simulink model "variant_3_MRC_SimulationModel"  (R2015b)
settings: Solver=ode3  SolverMode=SingleTasking  StartTime=0.0  StopTime=inf  RelTol=1e-3
PreLoadFcn:
  | addLibrariesInPath('sim')
PostLoadFcn:
  | loadRobotParameters
StartFcn:
  | simApp = SimDisplay.getInstance;
  | simApp.reset;
  | simApp.TrackView.setup(double(SitesPositions), ObstaclesPositions,ObstaclesVertices,ObstaclesEdges);
undefined symbols (not defined in the file): AngularSpeed, AxleLength, do_one_run, EncL_init, EncR_init, EncRes, lcam, motorL, motorR, motorX, ObstaclesEdges, ObstaclesVertices, pcam, SitesPositions, startPos, TauMotor, theta0, Ts, WheelRadius
libraries: simulink x2, realtime_pacer_lib x1, cstblocks x1, simulink_extras x1
(part 2 of 3)

== stateflow chart variant_3_MRC_SimulationModel/InputProcessing/Brain ==
  state Mapping [parallel]
    settings: executionOrder=2
    state Gestion_Rien
      %Entrée dans cet état si la camera ni détecte ni cible ni obstacle
      %Entrée dans un des blocs suivant l'orientation du robot : Nord, Nord-Est,...
      %Les blocs devant le robot (dans le champ de vision de la caméra) sont mis à jour à rien
      entry:
      ajout_cible_nv=false;
      ajout_cible_v=false;
      fin=false;
      Coef_bord_x=0;
      Coef_bord_y=0;
      bord = false;
      state Nord_Est
        entry: %-22.5
        % 0.7 pour sin(45°)
        state Obstacle
          entry:
          Carte(Distance_max_x-1, Distance_max_y+1)=3;
        state Bord_gauche
          entry:
          Coef_bord_y=-2;
          %Coef_bord_x=0;
        state Bord_droit
          entry:
          Coef_bord_x=+2;
        state Distance
          entry:
          Distance_max_x=xy_carte(1)-round(distObsM/10)-1;
          Distance_max_y=xy_carte(2)+round(distObsM/10)+1;
        state x_max
          entry:
          Distance_max_x = 2;
        state y_max
          entry:
          Distance_max_y = 29;
        state Mise_a_jour_carte
          entry:
          Carte(xy_carte(1)-1, xy_carte(2)+1)=4;
          Carte(xy_carte(1)-2, xy_carte(2)+2)=4;
          Carte(Distance_max_x+1+Coef_bord_x:xy_carte(1)-3+Coef_bord_x, xy_carte(2)+3+Coef_bord_y:Distance_max_y-1+Coef_bord_y)=4;
        state Fin
          entry:
          fin=true;
        state Bord2
          entry:
          Carte(Distance_max_x:xy_carte(1)-3, Distance_max_y-3:Distance_max_y-2)=4;
          Carte(Distance_max_x+2:Distance_max_x+3, xy_carte(2)+3:Distance_max_y)=4;
        (default) -> Bord_gauche [order 2] : [orientation > -28]
        (default) -> Bord_droit [order 1] : [orientation < -62 ]
        (default) -> Distance [order 3] : [orientation <= -28 && orientation >= -62]
        Mise_a_jour_carte -> Obstacle [order 1] : [distObsM < 60 && bord]
        Obstacle -> Fin : [1]
        Bord_droit -> Distance
        Bord_gauche -> Distance
        Distance -> x_max [order 1] : [Distance_max_x < 2]
        Distance -> y_max [order 2] : [Distance_max_y > 29]
        Distance -> Mise_a_jour_carte [order 3] : [Distance_max_x > 1 && Distance_max_y < 30]
        y_max -> x_max [order 2] : [Distance_max_x < 2]
        x_max -> y_max [order 1] : [Distance_max_y > 29]
        y_max -> Mise_a_jour_carte [order 1] : [1]
        x_max -> Mise_a_jour_carte [order 2] : [1]
        Mise_a_jour_carte -> Bord2 [order 3] : [bord==false]
        Mise_a_jour_carte -> Fin [order 2] : [distObsM == 60 && bord]
        Bord2 -> Fin : [1]
      state Nord_Ouest
        state Bord_gauche1
          entry:
          Coef_bord_x=+2;
          bord = true;
        state Bord_droit1
          entry:
          Coef_bord_y=+2;
          bord=true;
        state Obstacle1
          entry:
          Carte(Distance_max_x-1, Distance_max_y-1)=3;
        state Distance1
          entry:
          Distance_max_x=xy_carte(1)-round(distObsM/10)-1;
          Distance_max_y=xy_carte(2)-round(distObsM/10)-1;
        state y_max1
          entry:
          Distance_max_y = 2;
        state x_max1
          entry:
          Distance_max_x = 2;
        state Mise_a_jour_carte1
          entry:
          Carte(xy_carte(1)-1, xy_carte(2)-1)=4;
          Carte(xy_carte(1)-2, xy_carte(2)-2)=4;
          Carte(Distance_max_x+1+Coef_bord_x:xy_carte(1)-3+Coef_bord_x, Distance_max_y+1+Coef_bord_y:xy_carte(2)-3+Coef_bord_y)=4;
        state Fin1
          entry:
          fin=true;
        state Bord1
          entry:
          Carte(Distance_max_x:xy_carte(1)+3, Distance_max_y+2:Distance_max_y+3)=4;
          Carte(Distance_max_x+2:Distance_max_x+3, Distance_max_y:xy_carte(2)+3)=4;
        (default) -> Mapping.Gestion_Rien.Nord_Ouest.Bord_gauche1 [order 1] : [orientation > -28]
        (default) -> Mapping.Gestion_Rien.Nord_Ouest.Bord_droit1 [order 2] : [orientation < -53 ]
        (default) -> Mapping.Gestion_Rien.Nord_Ouest.Distance1 [order 3] : [orientation <= -28 && orientation >= -53]
        Mapping.Gestion_Rien.Nord_Ouest.Bord_droit1 -> Mapping.Gestion_Rien.Nord_Ouest.Distance1
        Mapping.Gestion_Rien.Nord_Ouest.Bord_gauche1 -> Mapping.Gestion_Rien.Nord_Ouest.Distance1
        Mapping.Gestion_Rien.Nord_Ouest.Distance1 -> Mapping.Gestion_Rien.Nord_Ouest.x_max1 [order 1] : [Distance_max_x < 2]
        Mapping.Gestion_Rien.Nord_Ouest.Mise_a_jour_carte1 -> Mapping.Gestion_Rien.Nord_Ouest.Obstacle1 [order 1] : [distObsM < 60 && bord]
        Mapping.Gestion_Rien.Nord_Ouest.Obstacle1 -> Mapping.Gestion_Rien.Nord_Ouest.Fin1 : [1]
        Mapping.Gestion_Rien.Nord_Ouest.Distance1 -> Mapping.Gestion_Rien.Nord_Ouest.y_max1 [order 2] : [Distance_max_y < 2]
        Mapping.Gestion_Rien.Nord_Ouest.Distance1 -> Mapping.Gestion_Rien.Nord_Ouest.Mise_a_jour_carte1 [order 3] : [Distance_max_x > 1 && Distance_max_y > 1]
        Mapping.Gestion_Rien.Nord_Ouest.y_max1 -> Mapping.Gestion_Rien.Nord_Ouest.x_max1 [order 2] : [Distance_max_x < 2]
        Mapping.Gestion_Rien.Nord_Ouest.x_max1 -> Mapping.Gestion_Rien.Nord_Ouest.y_max1 [order 1] : [Distance_max_y < 2]
        Mapping.Gestion_Rien.Nord_Ouest.y_max1 -> Mapping.Gestion_Rien.Nord_Ouest.Mise_a_jour_carte1 [order 1] : [1]
        Mapping.Gestion_Rien.Nord_Ouest.x_max1 -> Mapping.Gestion_Rien.Nord_Ouest.Mise_a_jour_carte1 [order 2] : [1]
        Mapping.Gestion_Rien.Nord_Ouest.Mise_a_jour_carte1 -> Mapping.Gestion_Rien.Nord_Ouest.Bord1 [order 3] : [bord==false]
        Mapping.Gestion_Rien.Nord_Ouest.Mise_a_jour_carte1 -> Mapping.Gestion_Rien.Nord_Ouest.Fin1 [order 2] : [distObsM == 60 && bord]
        Mapping.Gestion_Rien.Nord_Ouest.Bord1 -> Mapping.Gestion_Rien.Nord_Ouest.Fin1 : [1]
      state Nord
        entry:
        state Distance2
          entry:
          Distance_max=xy_carte(1)-round(distObsM/10);
        state y_max2
          entry:
          Distance_max = 1;
        state Mise_a_jour_carte2
          entry:
          Carte(Distance_max:xy_carte(1), xy_carte(2))=4;
          Carte(Distance_max:xy_carte(1)-1, xy_carte(2)-1:xy_carte(2)+1)=4;
          Carte(Distance_max:xy_carte(1)-2, xy_carte(2)-2:xy_carte(2)+2)=4;
        state Obstacle2
          entry:
          Carte(Distance_max, xy_carte(2)-1:xy_carte(2)+1)=3;
        state Fin2
          entry:
          fin=true;
        (default) -> Mapping.Gestion_Rien.Nord.Distance2
        Mapping.Gestion_Rien.Nord.Distance2 -> Mapping.Gestion_Rien.Nord.y_max2 [order 1] : [Distance_max < 1]
        Mapping.Gestion_Rien.Nord.y_max2 -> Mapping.Gestion_Rien.Nord.Mise_a_jour_carte2 : [1]
        Mapping.Gestion_Rien.Nord.Distance2 -> Mapping.Gestion_Rien.Nord.Mise_a_jour_carte2 [order 2] : [Distance_max > 0]
        Mapping.Gestion_Rien.Nord.Mise_a_jour_carte2 -> Mapping.Gestion_Rien.Nord.Obstacle2 [order 1] : [distObsM < 60]
        Mapping.Gestion_Rien.Nord.Obstacle2 -> Mapping.Gestion_Rien.Nord.Fin2 : [1]
        Mapping.Gestion_Rien.Nord.Mise_a_jour_carte2 -> Mapping.Gestion_Rien.Nord.Fin2 [order 2] : [distObsM == 60]
      state Ouest
        state Distance2
          entry:
          Distance_max=xy_carte(2)-round(distObsM/10);
        state y_max2
          entry:
          Distance_max = 1;
        state Obstacle2
          entry:
          Carte(xy_carte(1)-1:xy_carte(1)+1, Distance_max)=3;
        state Mise_a_jour_carte2
          entry:
          Carte(xy_carte(1), Distance_max:xy_carte(2))=4;
          Carte(xy_carte(1)-1:xy_carte(1)+1, Distance_max:xy_carte(2)-1)=4;
          Carte(xy_carte(1)-2:xy_carte(1)+2, Distance_max:xy_carte(2)-3)=4;
        state Fin2
          entry:
          fin=true;
        (default) -> Mapping.Gestion_Rien.Ouest.Distance2
        Mapping.Gestion_Rien.Ouest.Distance2 -> Mapping.Gestion_Rien.Ouest.y_max2 [order 1] : [Distance_max < 1]
        Mapping.Gestion_Rien.Ouest.y_max2 -> Mapping.Gestion_Rien.Ouest.Mise_a_jour_carte2 : [1]
        Mapping.Gestion_Rien.Ouest.Distance2 -> Mapping.Gestion_Rien.Ouest.Mise_a_jour_carte2 [order 2] : [Distance_max > 0]
        Mapping.Gestion_Rien.Ouest.Mise_a_jour_carte2 -> Mapping.Gestion_Rien.Ouest.Obstacle2 [order 1] : [distObsM < 60]
        Mapping.Gestion_Rien.Ouest.Obstacle2 -> Mapping.Gestion_Rien.Ouest.Fin2 : [1]
        Mapping.Gestion_Rien.Ouest.Mise_a_jour_carte2 -> Mapping.Gestion_Rien.Ouest.Fin2 [order 2] : [distObsM == 60]
      state Est
        entry:
        state Distance1
          entry:
          Distance_max=xy_carte(2)+round(distObsM/10);
        state y_max1
          entry:
          Distance_max = 30;
        state Obstacle1
          entry:
          Carte(xy_carte(1)-1:xy_carte(1)+1, Distance_max)=3;
        state Mise_a_jour_carte1
          entry:
          Carte(xy_carte(1), xy_carte(2):Distance_max)=4;
          Carte(xy_carte(1)-1:xy_carte(1)+1, xy_carte(2)+1:Distance_max)=4;
          Carte(xy_carte(1)-2:xy_carte(1)+2, xy_carte(2)+3:Distance_max)=4;
        state Fin1
          entry:
          fin=true;
        (default) -> Mapping.Gestion_Rien.Est.Distance1
        Mapping.Gestion_Rien.Est.Distance1 -> Mapping.Gestion_Rien.Est.y_max1 [order 1] : [Distance_max > 30]
        Mapping.Gestion_Rien.Est.y_max1 -> Mapping.Gestion_Rien.Est.Mise_a_jour_carte1 : [1]
        Mapping.Gestion_Rien.Est.Distance1 -> Mapping.Gestion_Rien.Est.Mise_a_jour_carte1 [order 2] : [Distance_max < 31]
        Mapping.Gestion_Rien.Est.Mise_a_jour_carte1 -> Mapping.Gestion_Rien.Est.Obstacle1 [order 1] : [distObsM < 60]
        Mapping.Gestion_Rien.Est.Obstacle1 -> Mapping.Gestion_Rien.Est.Fin1 : [1]
        Mapping.Gestion_Rien.Est.Mise_a_jour_carte1 -> Mapping.Gestion_Rien.Est.Fin1 [order 2] : [distObsM == 60]
      state Sud
        entry:
        state Distance2
          entry:
          Distance_max=xy_carte(1)+round(distObsM/10);
        state y_max2
          entry:
          Distance_max = 30;
        state Obstacle2
          entry:
          Carte(Distance_max, xy_carte(2)-1:xy_carte(2)+1)=3;
        state Mise_a_jour_carte2
          entry:
          Carte(xy_carte(1):Distance_max, xy_carte(2))=4;
          Carte(xy_carte(1)+1:Distance_max, xy_carte(2)-1:xy_carte(2)+1)=4;
          Carte(xy_carte(1)+2:Distance_max, xy_carte(2)-2:xy_carte(2)+2)=4;
        state Fin2
          entry:
          fin=true;
        (default) -> Mapping.Gestion_Rien.Sud.Distance2
        Mapping.Gestion_Rien.Sud.Distance2 -> Mapping.Gestion_Rien.Sud.y_max2 [order 1] : [Distance_max > 30]
        Mapping.Gestion_Rien.Sud.y_max2 -> Mapping.Gestion_Rien.Sud.Mise_a_jour_carte2 : [1]
        Mapping.Gestion_Rien.Sud.Distance2 -> Mapping.Gestion_Rien.Sud.Mise_a_jour_carte2 [order 2] : [Distance_max < 31]
        Mapping.Gestion_Rien.Sud.Mise_a_jour_carte2 -> Mapping.Gestion_Rien.Sud.Obstacle2 [order 1] : [distObsM < 60]
        Mapping.Gestion_Rien.Sud.Obstacle2 -> Mapping.Gestion_Rien.Sud.Fin2 : [1]
        Mapping.Gestion_Rien.Sud.Mise_a_jour_carte2 -> Mapping.Gestion_Rien.Sud.Fin2 [order 2] : [distObsM == 60]
      state Sud_Ouest
        entry:
        state Bord_gauche2
          entry:
          Coef_bord_y=+2;
          bord=true;
        state Bord_droit2
          entry:
          Coef_bord_x=-2;
          bord=true;
        state Obstacle2
          entry:
          Carte(Distance_max_x+1, Distance_max_y-1)=3;
        state Distance2
          entry:
          Distance_max_x=xy_carte(1)+round(distObsM/10)+1;
          Distance_max_y=xy_carte(2)-round(distObsM/10)-1;
        state x_max2
          entry:
          Distance_max_x = 29;
        state y_max2
          entry:
          Distance_max_y = 2;
        state Mise_a_jour_carte2
          entry:
          Carte(xy_carte(1)+1, xy_carte(2)-1)=4;
          Carte(xy_carte(1)+2, xy_carte(2)-2)=4;
          Carte(xy_carte(1)+3+Coef_bord_x:Distance_max_x-1+Coef_bord_x, Distance_max_y+1+Coef_bord_y:xy_carte(2)-3+Coef_bord_y)=4;
        state Fin2
          entry:
          fin=true;
        state Bord1
          entry:
          Carte(xy_carte(1)+3:Distance_max_x, Distance_max_y-3:Distance_max_y-2)=4;
          Carte(Distance_max_x+2:Distance_max_x+3, Distance_max_y:xy_carte(2)-3)=4;
        (default) -> Bord_gauche2 [order 1] : [orientation > 98]
        (default) -> Bord_droit2 [order 2] : [orientation < 152 ]
        (default) -> Mapping.Gestion_Rien.Sud_Ouest.Distance2 [order 3] : [orientation <= 98 && orientation >= 152]
        Bord_droit2 -> Mapping.Gestion_Rien.Sud_Ouest.Distance2
        Bord_gauche2 -> Mapping.Gestion_Rien.Sud_Ouest.Distance2
        Mapping.Gestion_Rien.Sud_Ouest.Mise_a_jour_carte2 -> Mapping.Gestion_Rien.Sud_Ouest.Obstacle2 [order 1] : [distObsM < 60]
        Mapping.Gestion_Rien.Sud_Ouest.Obstacle2 -> Mapping.Gestion_Rien.Sud_Ouest.Fin2 : [1]
        Mapping.Gestion_Rien.Sud_Ouest.Distance2 -> x_max2 [order 1] : [Distance_max_x > 29]
        Mapping.Gestion_Rien.Sud_Ouest.Distance2 -> Mapping.Gestion_Rien.Sud_Ouest.y_max2 [order 2] : [Distance_max_y < 2]
        Mapping.Gestion_Rien.Sud_Ouest.Distance2 -> Mapping.Gestion_Rien.Sud_Ouest.Mise_a_jour_carte2 [order 3] : [Distance_max_x < 30 && Distance_max_y > 1]
        Mapping.Gestion_Rien.Sud_Ouest.y_max2 -> x_max2 [order 2] : [Distance_max_x > 29]
        Mapping.Gestion_Rien.Sud_Ouest.y_max2 -> Mapping.Gestion_Rien.Sud_Ouest.Mise_a_jour_carte2 [order 1] : [1]
        x_max2 -> Mapping.Gestion_Rien.Sud_Ouest.y_max2 [order 1] : [Distance_max_y < 2]
        x_max2 -> Mapping.Gestion_Rien.Sud_Ouest.Mise_a_jour_carte2 [order 2] : [1]
        Mapping.Gestion_Rien.Sud_Ouest.Bord1 -> Mapping.Gestion_Rien.Sud_Ouest.Fin2 : [1]
        Mapping.Gestion_Rien.Sud_Ouest.Mise_a_jour_carte2 -> Mapping.Gestion_Rien.Sud_Ouest.Fin2 [order 2] : [distObsM == 60 && bord]
        Mapping.Gestion_Rien.Sud_Ouest.Mise_a_jour_carte2 -> Mapping.Gestion_Rien.Sud_Ouest.Bord1 [order 3] : [bord==false]
      state Sud_Est
        entry:
        state Bord_gauche1
          entry:
          Coef_bord_x=-2;
          bord=true;
        state Bord_droit1
          entry:
          Coef_bord_y=-2;
          bord=true;
        state Distance1
          entry:
          Distance_max_x=xy_carte(1)+round(distObsM/10)+1;
          Distance_max_y=xy_carte(2)+round(distObsM/10)+1;
        state x_max1
          entry:
          Distance_max_x = 29;
        state y_max1
          entry:
          Distance_max_y = 29;
        state Obstacle1
          entry:
          Carte(Distance_max_x+1, Distance_max_y+1)=3;
        state Mise_a_jour_carte1
          entry:
          Carte(xy_carte(1)+1, xy_carte(2)+1)=4;
          Carte(xy_carte(1)+2, xy_carte(2)+2)=4;
          Carte(xy_carte(1)+3+Coef_bord_x:Distance_max_x-1+Coef_bord_x, xy_carte(2)+3+Coef_bord_y:Distance_max_y-1+Coef_bord_y)=4;
        state Fin1
          entry:
          fin=true;
        state Bord
          entry:
          Carte(xy_carte(1)+3:Distance_max_x, Distance_max_y-3:Distance_max_y-2)=4;
          Carte(Distance_max_x-3:Distance_max_x-2, xy_carte(2)+3:Distance_max_y)=4;
        (default) -> Mapping.Gestion_Rien.Sud_Est.Bord_gauche1 [order 2] : [orientation > -98]
        (default) -> Mapping.Gestion_Rien.Sud_Est.Bord_droit1 [order 3] : [orientation < -152 ]
        (default) -> Mapping.Gestion_Rien.Sud_Est.Distance1 [order 1] : [orientation <= -98 && orientation >= -152]
        Mapping.Gestion_Rien.Sud_Est.Bord_droit1 -> Mapping.Gestion_Rien.Sud_Est.Distance1
        Mapping.Gestion_Rien.Sud_Est.Bord_gauche1 -> Mapping.Gestion_Rien.Sud_Est.Distance1
        Mapping.Gestion_Rien.Sud_Est.Distance1 -> Mapping.Gestion_Rien.Sud_Est.x_max1 [order 1] : [Distance_max_x > 29]
        Mapping.Gestion_Rien.Sud_Est.Distance1 -> Mapping.Gestion_Rien.Sud_Est.y_max1 [order 2] : [Distance_max_y > 29]
        Mapping.Gestion_Rien.Sud_Est.Distance1 -> Mapping.Gestion_Rien.Sud_Est.Mise_a_jour_carte1 [order 3] : [Distance_max_x < 30 && Distance_max_y < 30]
        Mapping.Gestion_Rien.Sud_Est.x_max1 -> Mapping.Gestion_Rien.Sud_Est.y_max1 [order 1] : [Distance_max_y > 29]
        Mapping.Gestion_Rien.Sud_Est.y_max1 -> Mapping.Gestion_Rien.Sud_Est.Mise_a_jour_carte1 [order 1] : [1]
        Mapping.Gestion_Rien.Sud_Est.y_max1 -> Mapping.Gestion_Rien.Sud_Est.x_max1 [order 2] : [Distance_max_x > 29]
        Mapping.Gestion_Rien.Sud_Est.Mise_a_jour_carte1 -> Mapping.Gestion_Rien.Sud_Est.Obstacle1 [order 1] : [distObsM < 60]
        Mapping.Gestion_Rien.Sud_Est.x_max1 -> Mapping.Gestion_Rien.Sud_Est.Mise_a_jour_carte1 [order 2] : [1]
        Mapping.Gestion_Rien.Sud_Est.Obstacle1 -> Mapping.Gestion_Rien.Sud_Est.Fin1 : [1]
        Mapping.Gestion_Rien.Sud_Est.Mise_a_jour_carte1 -> Bord [order 3] : [bord==false]
        Mapping.Gestion_Rien.Sud_Est.Mise_a_jour_carte1 -> Mapping.Gestion_Rien.Sud_Est.Fin1 [order 2] : [distObsM == 60 && bord]
        Bord -> Mapping.Gestion_Rien.Sud_Est.Fin1 : [1]
      (default) -> Nord [order 1] : [(orientation>-18) && (orientation < 18)]
      (default) -> Nord_Ouest [order 8] : [(orientation>=18) && (orientation <= 72)]
      (default) -> Nord_Est [order 2] : [(orientation >=-72) && (orientation <= -18)]
      (default) -> Est [order 3] : [(orientation>-108) && (orientation < -72)]
      (default) -> Ouest [order 4] : [(orientation>72) && (orientation < 108)]
      (default) -> Sud_Ouest [order 7] : [(orientation>=108) && (orientation <= 162)]
      (default) -> Sud [order 6] : [(orientation>162) || (orientation < -162)]
      (default) -> Sud_Est [order 5] : [(orientation >= -162) && (orientation <= -108)]
    state init
      entry:
      % Initialisation de la carte : dimension : 30*30
      Carte=zeros(30,30); % Init à Inconnu
      % Initialisations des bords de la carte à obstacle
      Carte(:,1)=zeros(30,1)+3;
      Carte(:,30)=zeros(30,1)+3;
      Carte(1,:)=zeros(30,1)+3;
      Carte(30,:)=zeros(30,1)+3;
      % Initialisation de la position de départ à rien
      Carte(25,5)=4
      % Code :
      % 0 : Inconnu
      % 1 : Cible non visitée
      % 2 : Cible visitée
      % 3 : Obstacle
      % 4 : Rien
    state X_moins
      entry:
      Carte(2:xy_carte(1), xy_carte(2))=4;
    state Y_moins
      entry:
      Carte(xy_carte(1), 2:xy_carte(2))=4;
    state X_plus
      entry:
      Carte(xy_carte(1):29, xy_carte(2))=4;
    state Y_plus
      entry:
      Carte(xy_carte(1), xy_carte(2):29)=4;
    state XY_moins
      entry:
      Carte(2:xy_carte(1), 2:xy_carte(2))=4;
    state XY_moins1
      entry:
      Carte(xy_carte(1):29, xy_carte(2):29)=4;
    state Ajout_cible_non_visitee
      entry:
      Carte(30-round(cible_en_vue(2)/10), round(cible_en_vue(1)/10)) = 1;
    state Ajout_cible_visitee
      entry:
      %Carte(30-round(cible(2,num_cible)/10), round(cible(1,num_cible)/10)) = 2;
      Carte(xy_carte(1),xy_carte(2))=2;
    (default) -> Mapping.init
    Mapping.init -> Gestion_Rien : [1]
    Gestion_Rien -> Gestion_Rien [order 5] : [~ajout_cible_nv && ~ajout_cible_v && fin && xy_carte(1) >= 4 && xy_carte(2) >= 4 ...
        | && xy_carte(1) <= 26 && xy_carte(2) <= 26]
    Gestion_Rien -> X_moins [order 9] : [xy_carte(1) < 4]
    XY_moins -> X_moins [order 3] : [xy_carte(2) >= 4]
    X_moins -> Gestion_Rien : [xy_carte(1) >= 4]
    Gestion_Rien -> Y_moins [order 7] : [xy_carte(2) < 4]
    XY_moins -> Y_moins [order 2] : [xy_carte(1) >= 4]
    Y_moins -> Gestion_Rien : [xy_carte(2) >= 4]
    Gestion_Rien -> X_plus [order 8] : [xy_carte(1) > 26]
    XY_moins1 -> X_plus [order 3] : [xy_carte(2) <= 26]
    X_plus -> Gestion_Rien : [xy_carte(1)<=26]
    Gestion_Rien -> Y_plus [order 6] : [xy_carte(2) > 26]
    XY_moins1 -> Y_plus [order 2] : [xy_carte(1) <= 26]
    Y_plus -> Gestion_Rien : [xy_carte(2) <= 26]
    Gestion_Rien -> XY_moins [order 4] : [xy_carte(2) < 4 && xy_carte(1) < 4]
    XY_moins -> Gestion_Rien [order 1] : [xy_carte(2) >= 4 && xy_carte(1) >= 4]
    Gestion_Rien -> XY_moins1 [order 3] : [xy_carte(2) >26 && xy_carte(1) > 26]
    XY_moins1 -> Gestion_Rien [order 1] : [xy_carte(2) <= 26 && xy_carte(1) <= 26]
    Gestion_Rien -> Ajout_cible_non_visitee [order 1] : [ajout_cible_nv]
    Ajout_cible_non_visitee -> Gestion_Rien : [1]
    Ajout_cible_visitee -> Gestion_Rien : [1]
    Gestion_Rien -> Ajout_cible_visitee [order 2] : [ajout_cible_v]
  state condToStop =StopToTurn(quadrantD,quadrantF,signeA) [function]
    (default) -> (junction 1363)
    (junction 1363) -> (junction 1359) [order 4]
    (junction 1363) -> (junction 1376) [order 1] : [quadrantD==4]
    (junction 1363) -> (junction 1390) [order 3] : [quadrantD==2]
    (junction 1363) -> (junction 1318) [order 2] : [quadrantD==1]
    (junction 1376) -> (junction 1326) [order 1] : [quadrantF==4]
    (junction 1318) -> (junction 1514) [order 1] : [quadrantF==3]
    (junction 1376) -> (junction 1130) [order 4]
    (junction 1318) -> (junction 1452) [order 4]
    (junction 1376) -> (junction 1151) [order 2] : [quadrantF==1]
    (junction 1318) -> (junction 1523) [order 2] : [quadrantF==4]
    (junction 1376) -> (junction 1411) [order 3] : [quadrantF==2]
    (junction 1318) -> (junction 1354) [order 3] : [quadrantF==1]
    (junction 1359) -> (junction 1459) [order 1] : [quadrantF==1]
    (junction 1359) -> (junction 1458) [order 4]
    (junction 1359) -> (junction 1517) [order 2] : [quadrantF==4]
    (junction 1390) -> (junction 1399) [order 1] : [quadrantF==4]
    (junction 1390) -> (junction 1421) [order 4]
    (junction 1359) -> (junction 1451) [order 3] : [quadrantF==3]
    (junction 1390) -> (junction 1340) [order 2] : [quadrantF==1]
    (junction 1390) -> (junction 1528) [order 3] : [quadrantF==2]
    (junction 1411) -> (junction 1188) [order 2]
    (junction 1354) -> (junction 1495) [order 2]
    (junction 1326) -> (junction 1520) [order 1] : [signeA==1]
    (junction 1514) -> (junction 1396) [order 1] : [signeA==1]
    (junction 1411) -> (junction 1350) [order 1] : [signeA==1]
    (junction 1354) -> (junction 1327) [order 1] : [signeA==1]
    (junction 1326) -> (junction 1454) [order 2]
    (junction 1514) -> (junction 1432) [order 2]
    (junction 1151) -> (junction 1478) : {condToStop=2;}
    (junction 1130) -> (junction 1337) : {condToStop=1;}
    (junction 1523) -> (junction 1362) : {condToStop=1;}
    (junction 1452) -> (junction 1409) : {condToStop=2;}
    (junction 1451) -> (junction 1191) [order 2]
    (junction 1459) -> (junction 1391) [order 1] : [signeA==1]
    (junction 1451) -> (junction 1494) [order 1] : [signeA==1]
    (junction 1459) -> (junction 1128) [order 2]
    (junction 1517) -> (junction 1392) : {condToStop=2;}
    (junction 1458) -> (junction 1336) : {condToStop=3;}
    (junction 1528) -> (junction 1335) [order 2]
    (junction 1399) -> (junction 1164) [order 1] : [signeA==1]
    (junction 1528) -> (junction 1502) [order 1] : [signeA==1]
    (junction 1399) -> (junction 1488) [order 2]
    (junction 1340) -> (junction 1445) : {condToStop=1;}
    (junction 1421) -> (junction 1308) : {condToStop=4;}
    (junction 1520) -> (junction 1472) : {condToStop=1;}
    (junction 1350) -> (junction 1170) : {condToStop=3;}
    (junction 1188) -> (junction 1329) : {condToStop=2;}
    (junction 1396) -> (junction 1526) : {condToStop=1;}
    (junction 1327) -> (junction 1169) : {condToStop=1;}
    (junction 1495) -> (junction 1507) : {condToStop=2;}
    (junction 1454) -> (junction 1131) : {condToStop=2;}
    (junction 1432) -> (junction 1119) : {condToStop=4;}
    (junction 1391) -> (junction 1497) : {condToStop=3;}
    (junction 1494) -> (junction 1374) : {condToStop=1;}
    (junction 1191) -> (junction 1174) : {condToStop=2;}
    (junction 1128) -> (junction 1491) : {condToStop=2;}
    (junction 1164) -> (junction 1140) : {condToStop=1;}
    (junction 1502) -> (junction 1165) : {condToStop=1;}
    (junction 1335) -> (junction 1156) : {condToStop=2;}
    (junction 1488) -> (junction 1435) : {condToStop=4;}
  state GoTo [parallel]
    settings: executionOrder=4
    state To
      entry:
      Cmd.Mode = EMode.SPEED;
      Cmd.Angle=single(0);
      Cmd.Position=single(0);
      if ((Target==3 || Target==4 || Target==5) && next)
      xyf=cible_en_vue
      else
      xyf=[(I_col*10);(300-I_row*10)]
      end
      %xyfp=xyf;
      xyi=[xy(1);xy(2)];
      distance=sqrt((xyf(2)-xy(2))^2+(xyf(1)-xy(1))^2);
      orientationI=orientation;
      angle=acosd(abs(xyf(2)-xy(2))/distance);
      v=0;
      (default) -> (junction 1146)
      (junction 1146) -> (junction 1189) [order 2]
      (junction 1189) -> (junction 1173) [order 1] : [xyf(1)>=xy(1)]
      (junction 1146) -> (junction 1313) [order 1] : [xyf(2)>=xy(2)]
      (junction 1189) -> (junction 1324) [order 2] : {anglef=180-angle;}%quadrant II
      (junction 1173) -> (junction 1510) : {anglef=-(180-angle);}%quadrant III
      (junction 1324) -> (junction 1510)
      (junction 1510) -> (junction 1518)
      (junction 1313) -> (junction 1135) [order 1] : [xyf(1)>xy(1)]
      (junction 1313) -> (junction 1430) [order 2] : {anglef=angle;}%quadrant I
      (junction 1135) -> (junction 1518) : {anglef=-angle;} %quadrant IV
      (junction 1518) -> (junction 1430)
      (junction 1430) -> (junction 1310) : {angleafaire=orientationI-anglef;}
      (junction 1310) -> (junction 1476) [order 1] : [angleafaire>180]
      (junction 1476) -> (junction 1333) : {angleafaire=angleafaire-360;}
      (junction 1333) -> (junction 1408)
      (junction 1310) -> (junction 1300) [order 2]
      (junction 1300) -> (junction 1439) [order 1] : [angleafaire<-180]
      (junction 1439) -> (junction 1408) : {angleafaire=angleafaire+360;}
      (junction 1408) -> (junction 1414)
      (junction 1300) -> (junction 1414) [order 2]
      (junction 1414) -> (junction 1410) : {[orientationF,orientationF360]=CalculateAngle(orientationI-angleafaire);
          | quadD=DetQuad(orientation360);
          | quadF=DetQuad(orientationF360);
          | signeAngle=sign(angleafaire);
          | conditionToStop=StopToTurn(quadD,quadF,signeAngle);
          | DoAngle(angleafaire);}
    state init
      entry:
      Cmd.Mode = EMode.SPEED; % Speed control
      Cmd.Angle=single(0);
      Cmd.Position=single(0);
      Obstacle=0;
      I_row=0;
      I_col=30;
      Target=0;
    state Attente1 [commented out]
      entry:
      GoTo_End = 1;
    state Accel
      entry:
      Cmd.Mode = EMode.SPEED;
      Cmd.Angle=single(0);
      d=sqrt((xyi(2)-xy(2))^2+(xyi(1)-xy(1))^2); %distance parcourue
      (junction 1380) -> (junction 1400) [order 2] : [d<40]
      (junction 1400) -> (junction 1397) : {v=20;}
      (junction 1380) -> (junction 1386) [order 3] : [d<30]
      (junction 1386) -> (junction 1397) : {v=50;}
      (default) -> (junction 1315)
      (junction 1380) -> (junction 1367) [order 4] : [d<10]
      (junction 1367) -> (junction 1397) : {v=10;}
      (junction 1380) -> (junction 1416) [order 1] : [d>distance-3]
      (junction 1416) -> (junction 1397) : {v=0;}
      (junction 1315) -> (junction 1380) [order 1] : [distance<50]
      (junction 1397) -> (junction 1521)
      (junction 1315) -> (junction 1355) [order 2]
      (junction 1355) -> (junction 1152) [order 1] : [d<50]
      (junction 1152) -> (junction 1521) : {v=v+10;}
      (junction 1355) -> (junction 1469) [order 2]
      (junction 1521) -> (junction 1434)
      (junction 1303) -> (junction 1434) : {v=50;}
      (junction 1469) -> (junction 1303) [order 1] : [d<distance-50]
      (junction 1434) -> (junction 1448)
      (junction 1469) -> (junction 1379) [order 2]
      (junction 1379) -> (junction 1470) [order 1] : [d<distance-30]
      (junction 1470) -> (junction 1312) [order 1] : [v>10]
      (junction 1312) -> (junction 1448) : {v=v-10;}
      (junction 1470) -> (junction 1381) [order 2]
      (junction 1379) -> (junction 1450) [order 2]
      (junction 1448) -> (junction 1388)
      (junction 1450) -> (junction 1126) [order 1] : [d<distance-10]
      (junction 1126) -> (junction 1388) : {v=5;}
      (junction 1450) -> (junction 1345) [order 2] : {Cmd.Position=single(0);
          | v=0;}
      (junction 1388) -> (junction 1381)
      (junction 1381) -> (junction 1345) : {Cmd.Position=single(v);}
    state Attente
      entry:
      disp('attente_redemarre')
    state Tourne
      entry:
      disp('attente_tourne')
      Cmd.Mode = EMode.SPEED;
      Cmd.Angle=single(0);
    (default) -> GoTo.init
    GoTo.init -> To : after(0.2,sec)
    Attente1 -> To [commented out] : [(xyf(1) ~= xyfp(1)) || (xyf(2) ~= xyfp(2))]
    Accel -> To [order 4] : [v==0]
    Accel -> Attente1 [commented out] : [v == 0]
    To -> GoTo.Attente [order 2] : [Target==1 || Target==5]
    To -> GoTo.Attente [order 1] : [(Obstacle==1) || (Obstacle==2)]
    Accel -> GoTo.Attente [order 1] : [(Obstacle==1) || (Obstacle==2)]
    GoTo.Attente -> To [order 1] : [Target~=1 && Obstacle==0]
    Accel -> GoTo.Attente [order 2] : [Target==1 || Target==5]
    GoTo.Attente -> To [order 2] : [Target==0 && Obstacle==0]
    Accel -> Accel [order 3] : after(0.2,sec)
    To -> Tourne [order 3] : [(conditionToStop==2 && orientation>=orientationF)...
        |  || (conditionToStop==1 && orientation<=orientationF) ...
        | || (conditionToStop==3 && orientation360<=orientationF)...
        |  || (conditionToStop==4 && orientation360>=orientationF360)...
        | || (Robot.Distance(1) ~= 0 && Target==2)]
    Tourne -> Accel : [Target==0  && Obstacle==0]
    To -> Accel [commented out] : [(conditionToStop==2 && orientation>=orientationF)...
        |  || (conditionToStop==1 && orientation<=orientationF) ...
        | || (conditionToStop==3 && orientation360<=orientationF)...
        |  || (conditionToStop==4 && orientation360>=orientationF360)]
  state Test_GoTo1 [parallel] [commented out]
    state a0 [commented out]
      entry:
      GoTo_End = 0;
      xyf=[250;150]
    state a1 [commented out]
      entry:
      GoTo_End = 0;
      xyf=[100;100]
    state a01 [commented out]
      entry:
      GoTo_End = 0;
      xyf=[90;50]
    state a2 [commented out]
      entry:
      GoTo_End = 0;
      xyf=[275;150]
    state a3 [commented out]
      entry:
      GoTo_End = 0;
      xyf=[250;50]
    (default) -> a0 [commented out]
    a0 -> a1 [commented out] : [GoTo_End == 1]
    a1 -> a01 [commented out] : [GoTo_End == 1]
    a01 -> a2 [commented out] : [GoTo_End == 1]
    a2 -> a3 [commented out] : [GoTo_End == 1]
  state quadrant=DetQuad(angle_orientation) [function]
    (default) -> (junction 1239)
    (junction 1239) -> (junction 1238) [order 1] : [angle_orientation<=90]
    (junction 1238) -> (junction 1237) : {quadrant=1;}
    (junction 1239) -> (junction 1236) [order 2]
    (junction 1237) -> (junction 1242)
    (junction 1236) -> (junction 1235) [order 1] : [angle_orientation<=180]
    (junction 1235) -> (junction 1242) : {quadrant=2;}
    (junction 1236) -> (junction 1234) [order 2]
    (junction 1242) -> (junction 1250)
    (junction 1234) -> (junction 1251) [order 1] : [angle_orientation<=270]
    (junction 1251) -> (junction 1250) : {quadrant=3;}
    (junction 1250) -> (junction 1249)
    (junction 1234) -> (junction 1249) [order 2] : {quadrant=4;}
  state [oF,oF360]=CalculateAngle(angletocalculate) [function]
    (default) -> (junction 1254) : {oF360=angletocalculate;}
    (junction 1254) -> (junction 1272) [order 1] : [oF360>180]
    (junction 1272) -> (junction 1271) : {oF=oF360-360;}
    (junction 1271) -> (junction 1267)
    (junction 1254) -> (junction 1268) [order 2]
    (junction 1270) -> (junction 1269) [order 1] : [oF360<-180]
    (junction 1268) -> (junction 1270) [order 1] : [oF360<0]
    (junction 1269) -> (junction 1267) : {oF=oF360+360;
        | oF360=oF360+360;}
    (junction 1270) -> (junction 1273) [order 2] : {oF=oF360;
        | oF360=oF360+360;}
    (junction 1268) -> (junction 1266) [order 2] : {oF=oF360;}
  state DoAngle(angletodo) [function]
    (default) -> (junction 1274) : {%orientationI=orientation
        | %oF360=orientationI-angletodo
        | Cmd.Mode = EMode.SPEED;
        | Cmd.Position=single(0);
        | Cmd.Angle=single(50*sign(angletodo));
        | }
  state Brain [parallel]
    settings: executionOrder=7
    state Explore
      entry:
      Cmd.Mode = EMode.SPEED; % Speed control
      (default) -> (junction 1285)
      Explore -> (junction 1285) [order 1]
      (junction 1285) -> (junction 1202) [order 1] : [correction_status == EObstacles.AVOIDANCE]
      (junction 1285) -> (junction 1294) [order 2]
      (junction 1202) -> (junction 1288) : {
          | % Stop and turn
          | Obstacle=2;
          | }
      (junction 1294) -> (junction 1293) [order 1] : [correction_status == EObstacles.CORRECTION]
      (junction 1294) -> (junction 1292) [order 2]
      (junction 1293) -> (junction 1289) : {Obstacle=1;}
      (junction 1292) -> (junction 1291) [order 1] : [Target==4 || Target==5]
      (junction 1291) -> (junction 1289)
      (junction 1292) -> (junction 1290) [order 2] : {Target=0;}
      (junction 1289) -> (junction 1290)
      (junction 1288) -> (junction 1289)
      (junction 1290) -> (junction 1287)
    state TargetInView
      entry,during:
      if (Target==0 || Target==1 || Target==2)
      Target=1
      else
      Target=5
      end
      [~,ind] = min(Robot.Distance(1));
      TargetDistance = single(Robot.Distance(ind));
      TargetAngle = -single(Robot.Bearing(ind));
      Cmd.Mode = EMode.SPEED;
      Cmd.Angle = 0.7*TargetAngle;
      Cmd.Position=single(30);
    state Wait_for_scoring
      entry:
      Target=2
      ajout_cible_v=true;
      Cmd.Mode = EMode.SPEED;
      Cmd.Position = single(0);
      Cmd.Angle = single(0);
      num_cible=num_cible+1; %% construction matrice avec cibles
      cible(:,num_cible)=xy;
    state Attente2
      entry:
      disp('attente_redemarre_cible')
    state GoToTarget
      entry:
      Target=1
      disp('Je vais sur la cible !')
      Cmd.Mode = EMode.DISTANCE; % Distance control
      Cmd.Position=TargetDistance;
      Cmd.Angle = TargetAngle;
    (default) -> Explore
    Explore -> TargetInView [order 1] : [Robot.Distance(1) ~= 0]
    TargetInView -> Explore [order 2] : [Robot.Distance(1) == 0 || next]
    Wait_for_scoring -> Explore [order 2] : [after(3,sec)]
    Wait_for_scoring -> Explore [order 1] : [next]
    TargetInView -> Attente2 [order 1] : [(Obstacle==1) || ...
        | (Obstacle==2)]
    Attente2 -> TargetInView [order 1] : [Obstacle==0]
    GoToTarget -> Attente2 [order 1] : [(Obstacle==1) ||...
        |  (Obstacle==2)]
    Attente2 -> GoToTarget [order 2] : [Obstacle==0]
    GoToTarget -> Wait_for_scoring [order 2] : [Robot.Remaining.Distance < 5]
    TargetInView -> GoToTarget [order 3] : [TargetDistance < 35]
  state Position [parallel]
    settings: executionOrder=5
    state Actualisation
      entry:
      E=Robot.EncodersCount;
      TourRoue=double(E-Eprecedent) ;%% delta nb de tours effectués
      Eprecedent=E;
      dd=7*pi.*TourRoue/636 ;%%delta distance parcourue [dg;dd]
      dr=(dd(1)+dd(2))/2;
      dteta=atan((dd(2)-dd(1))/(16.5));
      dxy=[dr*cos(teta); dr*sin(teta)];
      xy=xy+dxy;
      % Position du robot dans le repère de la matrice Carte
      xy_carte=[30-round(xy(2)/10);round(xy(1)/10)];
      teta=teta+dteta;
      orientation360=teta*180/pi-90;
      % Orientation, en degré, du robot par rapport à la verticale
      % Verticale : 0°, droite : -90°, gauche : +90°
      %orientation=orientation+dteta*180/pi;
      [orientation,orientation360]=CalculateAngle(orientation360);
      %Target
    state Init
      entry :
      TourRoue=[0;0];
      dd=[0;0];
      xy=[50;50]; % position x y de départ
      xy_carte=[25;5];
      teta=0;
      cible=zeros(2,10);
      num_cible=0;
      Eprecedent=Robot.EncodersCount;
      % Orientation du robot
      orientation=-90; % vers la droite au départ
    (default) -> Position.Init
    Position.Actualisation -> Position.Actualisation : [1]
    Position.Init -> Position.Actualisation : [1]
  state Obs_Correct [parallel]
    settings: executionOrder=8
    state stop
      entry:
      ModeCorrection=1;
      Cmd.Mode = EMode.SPEED;
      Cmd.Position = single(0);
      Cmd.Angle = correction_sign * single(30);
    state init
      entry:
      ModeCorrection=0;
    state attente
      entry:
      Obstacle=0;
      ModeCorrection=0;
      if Target==3
      Target==4
      end
    state GoSlow
      entry:
      Cmd.Mode = EMode.SPEED;
      Cmd.Position = single(20);
      Cmd.Angle = single(0);
    (default) -> Obs_Correct.init
    Obs_Correct.init -> Obs_Correct.stop : [Obstacle==1  &&(ModeAvoidance==0)]
    Obs_Correct.attente -> Obs_Correct.stop : [(Obstacle==1) &&(ModeAvoidance==0)]
    Obs_Correct.stop -> Obs_Correct.GoSlow : after(1.5,sec)
    Obs_Correct.GoSlow -> Obs_Correct.attente : after(2,sec)
  state Obs_Correct1 [parallel]
    settings: executionOrder=9
    state stop
      entry:
      ModeAvoidance=1;
      Cmd.Mode = EMode.SPEED;
      Cmd.Position = single(0);
      Cmd.Angle = correction_sign * single(30);
    state init
      entry:
      ModeAvoidance=0;
    state attente
      entry:
      Obstacle=0;
      ModeAvoidance=0;
      if Target==3
      Target==4
      end
    state GoSlow
      entry:
      Cmd.Mode = EMode.SPEED;
      Cmd.Position = single(10);
      Cmd.Angle = single(0);
    (default) -> Obs_Correct1.init
    Obs_Correct1.init -> Obs_Correct1.stop : [(Obstacle==2) && (ModeCorrection==0)]
    Obs_Correct1.attente -> Obs_Correct1.stop : [(Obstacle==2) && (ModeCorrection==0)]
    Obs_Correct1.stop -> Obs_Correct1.GoSlow : after(2,sec)
    Obs_Correct1.GoSlow -> Obs_Correct1.attente : after(3,sec)
  state Detection_distance [parallel]
    %Détection de la position d'une cible vue par la caméra
    settings: executionOrder=6
    state Actualisation
      state Depassement
        entry:
        (default) -> (junction 1508)
        (junction 1508) -> (junction 1527) [order 1] : [delta_x > 299]
        (junction 1316) -> (junction 1147) : {delta_y=1}
        (junction 1524) -> (junction 1147) [order 3]
        (junction 1524) -> (junction 1316) [order 1] : [delta_y<1]
        (junction 1527) -> (junction 1524) : {delta_x=299;}
        (junction 1508) -> (junction 1129) [order 2] : [delta_x<1]
        (junction 1508) -> (junction 1524) [order 3]
        (junction 1159) -> (junction 1147) : {delta_y=299}
        (junction 1129) -> (junction 1524) : {delta_x=1;}
        (junction 1524) -> (junction 1159) [order 2] : [delta_y>299]
      state Position_cible
        entry:
        dist_cible=double(Robot.Distance(1));
        ang_cible=double(Robot.Bearing(1));
        or=orientation;
        x=xy(1);
        y=xy(2);
        delta_y=y+dist_cible*cos((pi/180)*(ang_cible+or));
        delta_x=x+dist_cible*sin(-(pi/180)*(ang_cible+or));
      state Mise_a_jour
        entry:
        cible_en_vue=[delta_x;delta_y]
        Target=3
      state Recherche_si_cible_deja_vue
        entry:
        if (num_cible ~= 0) && (count_cible~=0)
        for i=1:10
        if ((cible_en_vue(1) < cible_estime(1,i)+20) && (cible_en_vue(1) > cible_estime(1,i)-20) ...
        && (cible_en_vue(2) < cible_estime(2,i)+20) &&(cible_en_vue(2) > cible_estime(2,i)-20))
        disp('Cible en vue déjà vue')
        vue = true;
        break
        end
        end
        end
      state Ajout_cible
        entry:
        ajout_cible_nv=true;
        count_cible = count_cible + 1;
        cible_estime(1:2,count_cible)=cible_en_vue;
      state Recherche_si_cible_deja_visitee
        entry:
        if (num_cible ~= 0) && (count_cible~=0)
        for i=1:10
        if ((cible_en_vue(1) < cible(1,i)+20)&& (cible_en_vue(1) > cible(1,i)-20) ...
        && (cible_en_vue(2) < cible(2,i)+20)&& (cible_en_vue(2) > cible(2,i)-20))
        disp('Cible en vue déjà visitée. J y vais pas !')
        next = true;
        break
        end
        end
        end
      (default) -> Position_cible
      Position_cible -> Depassement
      Depassement -> Mise_a_jour
      Recherche_si_cible_deja_vue -> Ajout_cible [order 1] : [~vue]
      Mise_a_jour -> Recherche_si_cible_deja_vue
      Ajout_cible -> Recherche_si_cible_deja_visitee
      Recherche_si_cible_deja_vue -> Recherche_si_cible_deja_visitee [order 2] : [vue]
    state Init
      entry:
      cible_en_vue=zeros(2,1);
      cible_estime=zeros(2,10);
      count_cible=0;
      next=false;
      vue=false;
    state Attente
      entry:
      next=false;
      vue=false;
      disp('Attente')
    (default) -> Detection_distance.Init
    Detection_distance.Init -> Detection_distance.Actualisation : [Robot.Distance(1) ~= 0]
    Detection_distance.Actualisation -> Detection_distance.Attente : [Robot.Distance(1)==0]
    Detection_distance.Attente -> Detection_distance.Actualisation : [Robot.Distance(1) ~= 0]
  state Affichage_carte [parallel] [commented out]
    state Wait [commented out]
      entry:
      figure(2)
    state affichage [commented out]
      entry:
      coder.extrinsic('image')
      figure(2)
      image(Carte,'CDataMapping','scaled')
      %colorBar
    (default) -> Affichage_carte.Wait [commented out]
    Affichage_carte.Wait -> Affichage_carte.affichage [commented out] : [1]
    Affichage_carte.affichage -> Affichage_carte.affichage [commented out] : [1]
  state Affichage_relief [parallel]
    settings: executionOrder=3
    state Wait
    state affichage
      entry:
      coder.extrinsic('image')
      image(Relief,'CDataMapping','scaled')
      %Recherche du point le plus inconnu
      [M,I] = max(Relief(:));
      [I_row, I_col] = ind2sub(size(Relief),I);
    (default) -> Affichage_relief.Wait
    Affichage_relief.Wait -> Affichage_relief.affichage : [afficher_relief]
    Affichage_relief.affichage -> Affichage_relief.Wait : [1]
  state CarteRelief [parallel]
    settings: executionOrder=1
    state init
      entry:
      Relief=zeros(30,30);
      fin_boucle=false;
      count=0;
      afficher_relief=false;
    state importer_carte
      entry:
      for li=2:29
      for co=2:29
      if (Carte(li,co) == 0)
      Relief(li,co) = 1;
      end
      end
      end
    state Calcul_profondeur
      entry:
      while (~fin_boucle || count == 500)
      Relief_temp = Relief;
      fin_boucle=true;
      for l=2:29
      for c=2:29
      point=Relief(l,c);
      if ((point ~= 0) && ((Relief(l+1,c) == point) || (l+1==30)) && ((Relief(l-1,c) == point) || (l-1==1)) && ((Relief(l,c+1) == point) || (c+1==30)) && ((Relief(l,c-1) == point) || (c-1==1)))
      Relief_temp(l,c) = point + 1;
      fin_boucle=false;
      end
      end
      end
      count = count + 1;
      Relief=Relief_temp;
      end
      afficher_relief=true;
    CarteRelief.init -> importer_carte : [1]
    (default) -> CarteRelief.init
    importer_carte -> Calcul_profondeur : [1]
    Calcul_profondeur -> CarteRelief.init : [1]
  data: quadrantD function_input; quadrantF function_input; signeA function_input; condToStop function_output; quadrant function_output; angle_orientation function_input; angletocalculate function_input; oF function_output; oF360 function_output; angletodo function_input; Cmd output Bus: bus_Command; Robot input Bus: bus_Robot; correction_status input Enum: EObstacles; ind local; correction_sign input single; TargetDistance local single; TargetAngle local single; y local; x local; teta local; E local; Eprecedent local; dteta local; dr local double; cible local; num_cible local; TourRoue local; dxy local; xy local; dd local; next local; i local; cible_estime local; count_cible local; delta_y local; delta_x local; cible_en_vue local; orientation local; angle_cible local; vue local; Object local; Var local; fasle local; ajout_obstacle local; ajout_rien local; ajout_cible_nv local; ajout_cible_v local; n local; D local; Carte local; carte local; xy_carte local; distObsM input double; Distance_max local; Distance_max_x local; Distance_max_y local; fin local; Coef_bord_min local; Coef_bord_max local; Coef_bord local; Coef_bord_y local; Coef_bord_x local; bord local; orientationI local; angleafaire local; orientation360 local; xyf local; angle local; v local; distance local; anglef local; quadD local; quadF local; d local; xyi local; iter local; Obstacle local; orientationF360 local; orientationF local; conditionToStop local; signeAngle local; col local; Relief local; line local; niveau local; Relief_temp local; fin_boucle local; l local; c local; point local; count local; li local; co local; afficher_relief local; I_col local; I_row local; M local; I local; Target local; ModeCorrection local; ModeAvoidance local; dist_cible local; ang_cible local; or local

== stateflow chart variant_3_MRC_SimulationModel/RobotModel/Robot/Sensors Camera_Distance/Distance_sensor/Scanner ==
  state ScanDistance
    state Scanning
      state LookFront
        entry:
        ArmAngle = int8(0);
        exit:
        scanner_value(EPosition.MIDDLE) = ArmDist;
        scanner_status = EPosition.MIDDLE;
      state LookLeft
        entry:
        ArmAngle = int8(25);
        exit:
        scanner_value(EPosition.LEFT) = ArmDist;
        scanner_status = EPosition.LEFT;
      state LookRight
        entry:
        ArmAngle = int8(-25);
        exit:
        scanner_value(EPosition.RIGHT) = ArmDist;
        scanner_status = EPosition.RIGHT;
      (default) -> LookFront : {
          | scanner_value = int8(-1*ones(1,3));
          | scanner_status = EPosition.NO;
          | }
      LookLeft -> LookFront [order 1] : after(4,tick)
      LookLeft -> LookFront [order 2] : [after(3,tick) && ArmDist == -1]
      LookFront -> LookRight [order 1] : after(3,tick)
      LookFront -> LookRight [order 2] : [after(2,tick) && ArmDist == -1]
      LookRight -> LookLeft [order 1] : after(3,tick)
      LookRight -> LookLeft [order 2] : [after(2,tick) && ArmDist == -1]
    state Idle
      entry:
      ArmAngle = int8(0);
      during,exit:
      scanner_value = int8(-1*ones(1,3));
      scanner_status = EPosition.NO;
    (default) -> Scanning
    Scanning -> Idle : pauseScanner
    Idle -> Scanning : resumeScanner
  data: ArmDist input; scanner_status output Enum: EPosition; scanner_value output int8; ArmAngle output
  events: resumeScanner local FUNCTION_CALL_EVENT; pauseScanner local FUNCTION_CALL_EVENT

== stateflow chart variant_3_MRC_SimulationModel/RobotModel/Controller/FeedbackController/ControllerModesDistance ==
  state CurrentMove [parallel]
    settings: executionOrder=1
    state Normal
      entry:
      EncodersZero = Encoders;
      entry,during:
      CurrentDistance = CurrentMoveFcn(Encoders,EncodersZero);
    state distance = CurrentMoveFcn(enc,zero) [function]
    (default) -> Normal
    Normal -> Normal : Reset
  state ModeControl [parallel]
    settings: executionOrder=2
    state SpeedControl
      entry:
      CurrentMove.Reset;
      ResetDistancePI;
      DistanceError = Cmd.Position;
      PrevDistance = CurrentDistance;
      during:
      DistanceError = (Cmd.Position - (CurrentDistance-PrevDistance)/Ts);
      PrevDistance = CurrentDistance;
    state DistanceControl
      entry:
      CurrentMove.Reset;
      ResetDistancePI;
      entry,during:
      DistanceError = Cmd.Position - CurrentDistance;
    (default) -> (junction 73)
    (junction 73) -> (junction 72) [order 1] : [Cmd.Mode == EMode.SPEED]
    (junction 73) -> DistanceControl [order 2]
    (junction 72) -> SpeedControl
    SpeedControl -> DistanceControl : [Cmd.Mode == EMode.DISTANCE]
    DistanceControl -> SpeedControl : [Cmd.Mode == EMode.SPEED]
  state ResetIntegrator [parallel]
    settings: executionOrder=4
    (default) -> (junction 189) : {
        | PrevCmd = Cmd.Position;
        | PrevMode = Cmd.Mode;
        | }
    ResetIntegrator -> (junction 189)
    (junction 189) -> (junction 192) [order 1] : [Cmd.Mode ~= PrevMode]
    (junction 189) -> (junction 179) [order 2]
    (junction 192) -> (junction 185)
    (junction 179) -> (junction 185) [order 1] : [sign(Cmd.Position) ~= sign(PrevCmd)]
    (junction 179) -> (junction 188) [order 2]
    (junction 185) -> (junction 187) : {
        | ResetDistancePI;
        | }
    (junction 187) -> (junction 188)
    (junction 188) -> (junction 181) : {
        | PrevCmd = Cmd.Position;
        | PrevMode = Cmd.Mode;
        | }
  state ErrorInitialCondition [parallel]
    settings: executionOrder=3
    (default) -> (junction 170)
    ErrorInitialCondition -> (junction 170)
    (junction 170) -> (junction 171) [order 1] : [abs(DistanceError) < 30 && ...
        | abs(Cmd.Angle) < 1 && ...
        | Cmd.Mode == EMode.SPEED]
    (junction 170) -> (junction 172) [order 2] : {
        | DistanceIC = single(0);
        | }
    (junction 171) -> (junction 173) : {
        | DistanceIC = 30 * sign(Cmd.Position) - DistanceError;
        | }
    (junction 173) -> (junction 172)
    (junction 172) -> (junction 174)
  data: enc function_input int32 size=2; zero function_input int32 size=2; distance function_output; EncodersZero local int32 size=2; PrevDistance local; PrevCmd local; PrevMode local; Encoders input int32 size=2; CurrentDistance local single; DistanceError output single size=1; Cmd input Bus: bus_Command; Ts parameter; DistanceIC output
  events: Reset local FUNCTION_CALL_EVENT; ResetDistancePI output EITHER_EDGE_EVENT
